simulink model "sldemo_lct_gain"  (Simulink 7.6)
settings: Solver=FixedStepDiscrete  StartTime=0.0  StopTime=10.0  FixedStep=1  RelTol=1e-3
Description:
  | Return Arguments
settings Model: Creator=The MathWorks Inc.  ExtModeAutoUpdateStatusClock=off
settings DataIOCC: SaveOutput=off  SaveTime=off  SignalLoggingName=logsOut
settings OptimizationCC: InlineParams=on  InlineInvariantSignals=on  ZeroExternalMemoryAtStartup=off  ZeroInternalMemoryAtStartup=off  InitFltsAndDblsToZero=on  OptimizeModelRefInitCode=on  LifeSpan=1
settings DebuggingCC: SaveWithParameterizedLinksMsg=none  SignalResolutionControl=TryResolveAllWithWarning  SolverPrmCheckMsg=none  MultiTaskDSMMsg=warning  MultiTaskCondExecSysMsg=none
settings HardwareCC: TargetUnknown=on
settings RTWCC: SystemTargetFile=ert.tlc  GenCodeOnly=on  TemplateMakefile=ert_default_tmf  Description=RTW Embedded Coder (no auto configuration)  GenerateReport=on  ProcessScript=ert_make_rtw_hook  IncludeHyperlinkInReport=on  LaunchReport=on  IncludeERTFirstTime=on
settings CodeAppCC: IgnoreCustomStorageClasses=off
settings ERTTargetCC: TargetFcnLib=ansi_tfl_tmw.mat  MultiwordLength=2048  GenerateSampleERTMain=on  IncludeMdlTerminateFcn=off  SuppressErrorStatus=on  InlinedParameterPlacement=NonHierarchical  ERTSrcFileBannerTemplate=example_banner.tlc  ERTHdrFileBannerTemplate=example_banner.tlc  ERTCustomFileTemplate=example_file_process.tlc  ConvertIfToSwitch=off

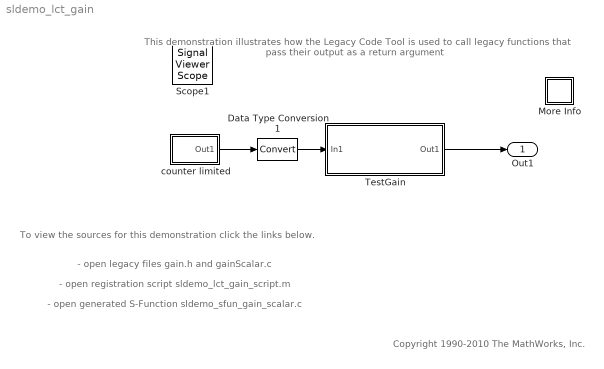
== system sldemo_lct_gain ==
  note: Copyright 1990-2010 The MathWorks, Inc.
  note: This demonstration illustrates how the Legacy Code Tool is used to
      | call legacy functions that pass their output as a return argument
  note: - open legacy files gain.h and gainScalar.c
  note: To view the sources for this demonstration
      | click the links below.
  note: - open registration script sldemo_lct_gain_script.m
  note: - open generated S-Function sldemo_sfun_gain_scalar.c
  Data Type Conversion1 : DataTypeConversion  RndMeth=Zero
  More Info : Subsystem
      settings: OpenFcn=showdemo('sldemo_lct_gain_script')
      mask Display: disp('?')
  TestGain : Subsystem
  counter limited : Subsystem  mask(CounterLimited){th=2^16-1}
      mask prompts: th "Threshold:"
  Out1 : Outport
  Scope1 : SignalViewerScope  IOType=viewer  RefreshTime=0.035000
      settings: YMin=0  YMax=120
  wires:
  TestGain/1(Out1) -> Out1/1
  counter limited/1(Out1) -> Data Type Conversion1/1
  Data Type Conversion1/1 -> TestGain/1(In1)

== system sldemo_lct_gain/More Info ==

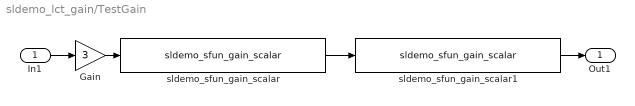
== system sldemo_lct_gain/TestGain ==
  In1 : Inport
  Gain : Gain  Gain=3  OutDataTypeStr=Inherit: Inherit via back propagation
  sldemo_sfun_gain_scalar : S-Function  FunctionName=sldemo_sfun_gain_scalar  Parameters=SParameter1  EnableBusSupport=off  mask(Legacy Function){SFunctionSpec=single y1 = gainScalar(single u1, single p1), SParameter1=single(2), ShowSpec=on}
      mask prompts: SParameter1 "P1:"; ShowSpec "Display function specification"
      mask help:
      | This block allows you to call the legacy functions specified by the following Legacy Code Tool definition:
      | def.SFunctionName = 'sldemo_sfun_gain_scalar';
      | def.OutputFcnSpec = 'single y1 = gainScalar(single u1, single p1)';
      | def.HeaderFiles = {'gain.h'};
      | def.SourceFiles = {'gainScalar.c'};
      | def.IncPaths = {'sldemo_lct_src'};
      | def.SrcPaths = {'sldemo_lct_src'};
      mask Help: <p>This block was generated automatically by the Legacy Code Tool. For detailed help on this tool, call<a href="matlab:legacy_code('help')"> legacy_code('help')</a>.</p>
      mask CallbackString:
      | ||if strcmp(get_param(gcbh, 'ShowSpec'), 'on')
      |   set_param(gcbh, 'MaskDisplay', sprintf('fprintf(''%s'');', get_param(gcbh, 'SFunctionSpec')));
      | else
      |   set_param(gcbh, 'MaskDisplay', sprintf('fprintf(''%s'');', get_param(gcbh, 'FunctionName')));
      | end
      mask Display: fprintf('single y1 = gainScalar(single u1, single p1)');
  sldemo_sfun_gain_scalar1 : S-Function  FunctionName=sldemo_sfun_gain_scalar  Parameters=SParameter1  EnableBusSupport=off  mask(Legacy Function){SFunctionSpec=single y1 = gainScalar(single u1, single p1), SParameter1=single(2), ShowSpec=on}
      mask prompts: SParameter1 "P1:"; ShowSpec "Display function specification"
      mask help:
      | This block allows you to call the legacy functions specified by the following Legacy Code Tool definition:
      | def.SFunctionName = 'sldemo_sfun_gain_scalar';
      | def.OutputFcnSpec = 'single y1 = gainScalar(single u1, single p1)';
      | def.HeaderFiles = {'gain.h'};
      | def.SourceFiles = {'gainScalar.c'};
      | def.IncPaths = {'sldemo_lct_src'};
      | def.SrcPaths = {'sldemo_lct_src'};
      mask Help: <p>This block was generated automatically by the Legacy Code Tool. For detailed help on this tool, call<a href="matlab:legacy_code('help')"> legacy_code('help')</a>.</p>
      mask CallbackString:
      | ||if strcmp(get_param(gcbh, 'ShowSpec'), 'on')
      |   set_param(gcbh, 'MaskDisplay', sprintf('fprintf(''%s'');', get_param(gcbh, 'SFunctionSpec')));
      | else
      |   set_param(gcbh, 'MaskDisplay', sprintf('fprintf(''%s'');', get_param(gcbh, 'FunctionName')));
      | end
      mask Display: fprintf('single y1 = gainScalar(single u1, single p1)');
  Out1 : Outport
  wires:
  Gain/1 -> sldemo_sfun_gain_scalar/1
  In1/1 -> Gain/1
  sldemo_sfun_gain_scalar/1 -> sldemo_sfun_gain_scalar1/1
  sldemo_sfun_gain_scalar1/1 -> Out1/1

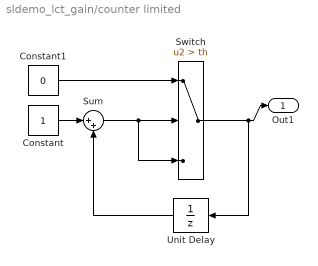
== system sldemo_lct_gain/counter limited ==
  Constant : Constant
  Constant1 : Constant  Value=0
  Sum : Sum  Inputs=|++
  Switch : Switch  Criteria=u2 > Threshold  Threshold=th  ZeroCross=off
  Unit Delay : UnitDelay  X0=-1  SampleTime=-1
  Out1 : Outport
  wires:
  Constant/1 -> Sum/1
  Sum/1 -> Switch/2, Switch/3
  Unit Delay/1 -> Sum/2
  Constant1/1 -> Switch/1
  Switch/1 -> Unit Delay/1, Out1/1
